simulink model "FixedWing_Model_nonlinearLQR_6_states"  (R2020b)
settings: Solver=VariableStepAuto  StartTime=0.0  StopTime=50  FixedStep=10^-4  RelTol=1e-7
values from neighbouring files (symbols this model uses):
  A_lat = [YB        Yp      -(u0-Yr)   g*cos(Theta0)   0;         A21       A22       A23        0             0;         A31       A32       A33        0             0;         0         1         0          0             0;         0         0         1          0             0]    [LQR_Dena_model_file_edited.m]
  A_long = [ Xu                    Xw              0              -g*cos(Theta0)            0;          Zu                    Zw              u0             -g*sin(Theta0)            0;          Mu+Mw_d*Zu            Mw+Mw_d*Zw      Mq+Mw_d*u0          0                    0;          0                     0               1                   0                    0;          -sin(Theta0)       -cos(Theta0)    ...(+51 chars)    [LQR_Dena_model_file_edited.m]
  b = 1.7    [LQR_Dena_model_file_edited.m]
  B_lat = [0        Ydr;        B21      B22;        B31      B32;        0        0;        0        0]    [LQR_Dena_model_file_edited.m]
  B_long = [ Xe         CXt;          Ze         0;          Me         0;          0          0;          0          0]    [LQR_Dena_model_file_edited.m]
  c = 0.28    [LQR_Dena_model_file_edited.m]
  C_lat = [0 0 0 1 0 ]    [LQR_Dena_model_file_edited.m]
  C_long = [0 0 0 1 0]    [LQR_Dena_model_file_edited.m]
  CL_aileron = 0.32935    [LQR_Dena_model_file_edited.m]
  CL_rudder = 0.003592    [LQR_Dena_model_file_edited.m]
  CLb = 0.029196    [LQR_Dena_model_file_edited.m]
  CLp = -0.44965    [LQR_Dena_model_file_edited.m]
  CLr = 0.0067709    [LQR_Dena_model_file_edited.m]
  CM_alpha = -0.1651    [LQR_Dena_model_file_edited.m]
  CM_alpha_dot = -6.5034    [LQR_Dena_model_file_edited.m]
  CMe = -1.3977    [LQR_Dena_model_file_edited.m]
  CMq = -11.7782    [LQR_Dena_model_file_edited.m]
  CMt = 0    [LQR_Dena_model_file_edited.m]
  CMu = 0.158*0    (= 0)    [LQR_Dena_model_file_edited.m]
  CN_aileron = 0.036215    [LQR_Dena_model_file_edited.m]
  CN_rudder = -0.045652    [LQR_Dena_model_file_edited.m]
  CNB = 0.066996    [LQR_Dena_model_file_edited.m]
  CNp = -0.030754    [LQR_Dena_model_file_edited.m]
  CNr = -0.064937    [LQR_Dena_model_file_edited.m]
  CX0 = -0.0094304    [LQR_Dena_model_file_edited.m]
  CX_alpha = (0.42565-0.21544)    (= 0.21021)    [LQR_Dena_model_file_edited.m]
  CXe = 0    [LQR_Dena_model_file_edited.m]
  CXt = 1    [LQR_Dena_model_file_edited.m]
  CXu = -(0.158*0)-0.0094304    (= -0.0094304)    [LQR_Dena_model_file_edited.m]
  CY_rudder = -0.10317    [LQR_Dena_model_file_edited.m]
  CYB = -0.16533    [LQR_Dena_model_file_edited.m]
  CYp = -0.00068802    [LQR_Dena_model_file_edited.m]
  CYr = 0.15502    [LQR_Dena_model_file_edited.m]
  CZ0 = -0.42565    [LQR_Dena_model_file_edited.m]
  CZ_alpha = -(4.8375+0.0094304)    (= -4.8469304)    [LQR_Dena_model_file_edited.m]
  CZ_alpha_dot = 1.3359    [LQR_Dena_model_file_edited.m]
  CZe = -0.56118    [LQR_Dena_model_file_edited.m]
  CZq = -7.3583    [LQR_Dena_model_file_edited.m]
  CZt = 0    [LQR_Dena_model_file_edited.m]
  CZu = -((0.052968^2)/(1-(0.052968)^2))*0.42565    (= -0.00119756738693)    [LQR_Dena_model_file_edited.m]
  d_aileron0 = 0    [LQR_Dena_model_file_edited.m]
  d_elevator0 = -0.6319*pi/180    (= -0.0110287355434)    [LQR_Dena_model_file_edited.m]
  D_long = zeros(5,2)    [LQR_Dena_model_file_edited.m]
  d_rudder0 = 0    [LQR_Dena_model_file_edited.m]
  d_Thrust0 = 5    [LQR_Dena_model_file_edited.m]
  e_longi = longd- [longi; 0]    [LQR_Dena_model_file_edited.m]
  Epsi0 = 0    [LQR_Dena_model_file_edited.m]
  Epsi_initial = Epsi0    (= 0)    [LQR_Dena_model_file_edited.m]
  g = 9.81    [LQR_Dena_model_file_edited.m]
  Hi = 120    [LQR_Dena_model_file_edited.m]
  Ix = 0.6465    [LQR_Dena_model_file_edited.m]
  Ixz = 0.0006584    [LQR_Dena_model_file_edited.m]
  Iy = 0.3048    [LQR_Dena_model_file_edited.m]
  Iz = 0.9359    [LQR_Dena_model_file_edited.m]
  K = K_long_hat(:,1:5)    [LQR_Dena_model_file_edited.m]
  K_lat_hat = lqr(A_lat_hat, B_lat_hat,Q_lat_hat,R_lat)    [LQR_Dena_model_file_edited.m]
  K_long = lqr(A_long, B_long,Q_long,R_long)    [LQR_Dena_model_file_edited.m]
  K_long_hat = lqr(A_long_hat, B_long_hat,Q_long_hat,R_long)    [LQR_Dena_model_file_edited.m]
  Ki = -K_long_hat(:,6)    [LQR_Dena_model_file_edited.m]
  lati = [ v_initial; p_initial; r_initial; Phi_initial; Epsi_initial]    [LQR_Dena_model_file_edited.m]
  longd = [u0; w0; q0; Theta0; Hi; 0]    [LQR_Dena_model_file_edited.m]
  longi = [ u_initial; w_initial; q_initial; Theta_initial; Ze0]    [LQR_Dena_model_file_edited.m]
  mass = 4    [LQR_Dena_model_file_edited.m]
  p0 = 0    [LQR_Dena_model_file_edited.m]
  p_initial = 0    [LQR_Dena_model_file_edited.m]
  Phi0 = 0    [LQR_Dena_model_file_edited.m]
  Phi_initial = Phi0    (= 0)    [LQR_Dena_model_file_edited.m]
  q0 = 0    [LQR_Dena_model_file_edited.m]
  q_initial = 0    [LQR_Dena_model_file_edited.m]
  r0 = 0    [LQR_Dena_model_file_edited.m]
  r_initial = 0    [LQR_Dena_model_file_edited.m]
  S = 0.471    [LQR_Dena_model_file_edited.m]
  Theta0 = 5.1*pi/180    (= 0.0890117918517)    [LQR_Dena_model_file_edited.m]
  Theta_initial = Theta0+(2*pi/180)    (= 0.123918376892)    [LQR_Dena_model_file_edited.m]
  u0 = sqrt(V0^2/(1+(tan(Theta0))^2))    [LQR_Dena_model_file_edited.m]
  u_initial = u0    [LQR_Dena_model_file_edited.m]
  v0 = 0    [LQR_Dena_model_file_edited.m]
  v_initial = v0    (= 0)    [LQR_Dena_model_file_edited.m]
  w0 = u0*tan(Theta0)    [LQR_Dena_model_file_edited.m]
  w_initial = w0    [LQR_Dena_model_file_edited.m]
  X0 = mass*g*sin(Theta0)    [LQR_Dena_model_file_edited.m]
  Xe0 = 0    [LQR_Dena_model_file_edited.m]
  Y0 = -mass*g*cos(Theta0)*sin(Phi0)    [LQR_Dena_model_file_edited.m]
  Ye0 = 0    [LQR_Dena_model_file_edited.m]
  Z0 = -mass*g*cos(Theta0)*cos(Phi0)    [LQR_Dena_model_file_edited.m]
  Ze0 = 120    [LQR_Dena_model_file_edited.m]
undefined symbols (not defined in the file or in its folder): A_hat, B_hat, C_hat, K_alt, K_e, Meu_e, use, W_e
libraries: simulink_extras x39, dspindex x3, aerolibatmos2 x1, aerolibutil x1, sharedtransform x1
(part 2 of 2)

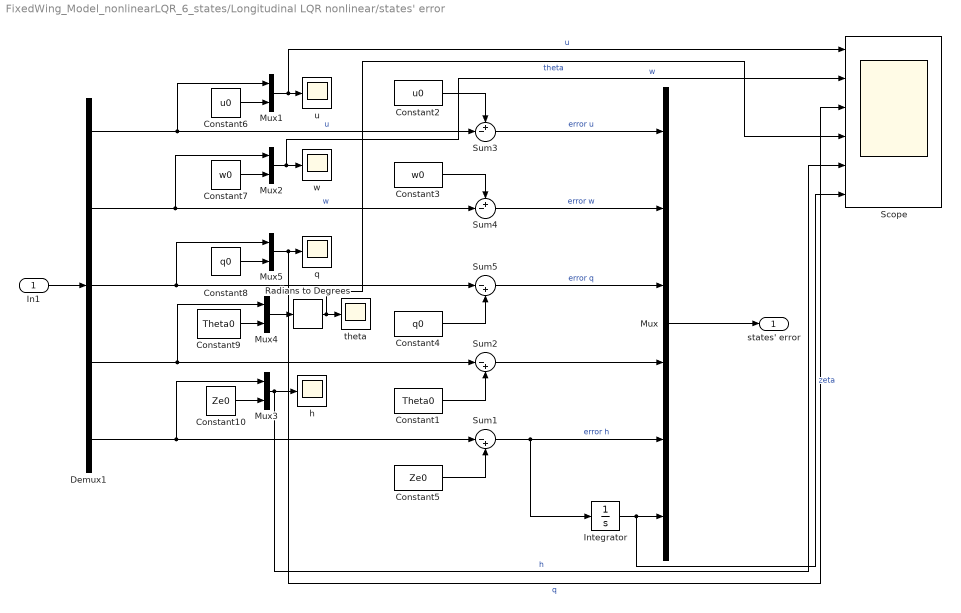
== system FixedWing_Model_nonlinearLQR_6_states/Longitudinal LQR nonlinear/states' error ==
  In1 : Inport
  Constant1 : Constant  Value=Theta0
  Constant10 : Constant  Value=Ze0
  Constant2 : Constant  Value=u0
  Constant3 : Constant  Value=w0
  Constant4 : Constant  Value=q0
  Constant5 : Constant  Value=Ze0
  Constant6 : Constant  Value=u0
  Constant7 : Constant  Value=w0
  Constant8 : Constant  Value=q0
  Constant9 : Constant  Value=Theta0
  Demux1 : Demux  Outputs=5
  Integrator : Integrator  InitialCondition=Ze0-Hi
  Mux : Mux  Inputs=6
  Mux{1..5} (5 alike) : Mux  Inputs=2
  Radians to Degrees : simulink_extras/Transformations/Radians to Degrees
  Scope : Scope  NumInputPorts=6
  Sum1 : Sum  Inputs=|-+
  Sum2 : Sum  Inputs=|-+
  Sum3 : Sum  Inputs=+-|
  Sum4 : Sum  Inputs=+-|
  Sum5 : Sum  Inputs=|-+
  h : Scope
  q : Scope
  theta : Scope
  u : Scope
  w : Scope
  states' error : Outport
  wires:
  Constant1/1 -> Sum2/2
  Constant4/1 -> Sum5/2
  Constant2/1 -> Sum3/1
  Sum3/1 -> Mux/1  "error u"
  Constant3/1 -> Sum4/1
  Sum4/1 -> Mux/2  "error w"
  In1/1 -> Demux1/1
  Sum5/1 -> Mux/3  "error q"
  Mux/1 -> states' error/1
  Constant5/1 -> Sum1/2
  Sum1/1 -> Mux/5, Integrator/1  "error h"
  Demux1/3 -> Mux5/1, Sum5/1
  Constant8/1 -> Mux5/2
  Constant9/1 -> Mux4/2
  Constant10/1 -> Mux3/2
  Constant7/1 -> Mux2/2
  Demux1/5 -> Mux3/1, Sum1/1
  Demux1/1 -> Mux1/1, Sum3/2  "u"
  Demux1/2 -> Mux2/1, Sum4/2  "w"
  Constant6/1 -> Mux1/2
  Mux1/1 -> Scope/1, u/1  "u"
  Mux2/1 -> Scope/2, w/1  "w"
  Mux5/1 -> Scope/3, q/1  "q"
  Mux3/1 -> Scope/5, h/1  "h"
  Demux1/4 -> Mux4/1, Sum2/1
  Mux4/1 -> Radians to Degrees/1
  Radians to Degrees/1 -> Scope/4, theta/1  "theta"
  Sum2/1 -> Mux/4
  Integrator/1 -> Scope/6, Mux/6  "zeta"

== system FixedWing_Model_nonlinearLQR_6_states/Longitudinal LQR nonlinear seperated/theta' error ==
  states : Inport
  Constant1 : Constant  Value=Theta0
  Constant10 : Constant  Value=Ze0
  Constant6 : Constant  Value=u0
  Constant7 : Constant  Value=w0
  Constant8 : Constant  Value=q0
  Constant9 : Constant  Value=Theta0
  Demux1 : Demux  Outputs=5
  Mux{1..4,6} (5 alike) : Mux  Inputs=2
  Radians to Degrees : simulink_extras/Transformations/Radians to Degrees
  Sum2 : Sum  Inputs=|-+
  h : Scope
  q : Scope
  theta : Scope
  u : Scope
  w : Scope
  theta' error : Outport
  wires:
  Constant1/1 -> Sum2/2
  states/1 -> Demux1/1
  Constant9/1 -> Mux4/2
  Demux1/4 -> Mux4/1, Sum2/1
  Mux4/1 -> Radians to Degrees/1
  Radians to Degrees/1 -> theta/1
  Sum2/1 -> theta' error/1
  Demux1/3 -> Mux6/1
  Mux2/1 -> w/1
  Mux3/1 -> h/1
  Demux1/1 -> Mux1/1
  Constant7/1 -> Mux2/2
  Constant8/1 -> Mux6/2
  Constant10/1 -> Mux3/2
  Mux1/1 -> u/1
  Mux6/1 -> q/1
  Demux1/5 -> Mux3/1
  Constant6/1 -> Mux1/2
  Demux1/2 -> Mux2/1

== system FixedWing_Model_nonlinearLQR_6_states/Non linear/Euler ==
  p : Inport
  q : Inport  Port=2
  r : Inport  Port=3
  Subsystem : Subsystem
  Subsystem1 : Subsystem
  Subsystem2 : Subsystem
  Phi : Outport
  Theta : Outport  Port=2
  epsi : Outport  Port=3
  wires:
  Subsystem1/1(Theta) -> Theta/1, [Theta]
  Subsystem2/1(epsi) -> epsi/1
  [q] -> Subsystem/2(q)
  Subsystem/1(Phi) -> Phi/1, [Phi]
  [Theta] -> Subsystem/3(Theta)
  [r] -> Subsystem1/2(r)
  [Phi] -> Subsystem1/3(Phi)
  [Theta] -> Subsystem2/3(Theta)
  [q] -> Subsystem2/2(q)
  p/1 -> [p]
  q/1 -> [q]
  r/1 -> [r]
  [p] -> Subsystem/1(p)
  [r] -> Subsystem/4(r)
  [q] -> Subsystem1/1(q)
  [r] -> Subsystem2/1(r)
  [Phi] -> Subsystem2/4(Phi)

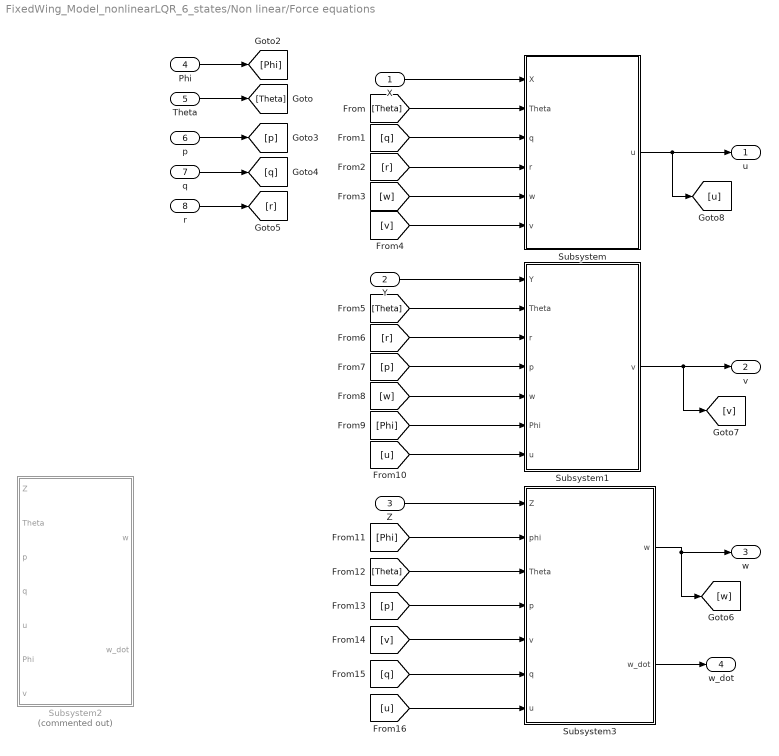
== system FixedWing_Model_nonlinearLQR_6_states/Non linear/Force equations ==
  X : Inport
  Y : Inport  Port=2
  Z : Inport  Port=3
  Phi : Inport  Port=4
  Theta : Inport  Port=5
  p : Inport  Port=6
  q : Inport  Port=7
  r : Inport  Port=8
  Subsystem : Subsystem
  Subsystem1 : Subsystem
  Subsystem2 : Subsystem  Commented=on
  Subsystem3 : Subsystem
  u : Outport
  v : Outport  Port=2
  w : Outport  Port=3
  w_dot : Outport  Port=4
  wires:
  Theta/1 -> [Theta]
  Phi/1 -> [Phi]
  p/1 -> [p]
  q/1 -> [q]
  r/1 -> [r]
  X/1 -> Subsystem/1(X)
  Y/1 -> Subsystem1/1(Y)
  Z/1 -> Subsystem3/1(Z)
  Subsystem/1(u) -> [u], u/1
  Subsystem1/1(v) -> v/1, [v]
  [Theta] -> Subsystem/2(Theta)
  [q] -> Subsystem/3(q)
  [r] -> Subsystem/4(r)
  [w] -> Subsystem/5(w)
  [v] -> Subsystem/6(v)
  [Theta] -> Subsystem1/2(Theta)
  [r] -> Subsystem1/3(r)
  [p] -> Subsystem1/4(p)
  [w] -> Subsystem1/5(w)
  [Phi] -> Subsystem1/6(Phi)
  [u] -> Subsystem1/7(u)
  [Phi] -> Subsystem3/2(phi)
  [p] -> Subsystem3/4(p)
  [v] -> Subsystem3/5(v)
  [q] -> Subsystem3/6(q)
  [u] -> Subsystem3/7(u)
  Subsystem3/1(w) -> [w], w/1
  Subsystem3/2(w_dot) -> w_dot/1
  [Theta] -> Subsystem3/3(Theta)

== system FixedWing_Model_nonlinearLQR_6_states/Non linear/Moment equations ==
  L : Inport
  M : Inport  Port=2
  N : Inport  Port=3
  Integrator : Integrator  InitialCondition=p_initial
  Integrator2 : Integrator  InitialCondition=r_initial
  Subsystem : Subsystem
  Subsystem1 : Subsystem
  Subsystem2 : Subsystem
  p : Outport
  q : Outport  Port=2
  r : Outport  Port=3
  wires:
  L/1 -> Subsystem/1(L)
  [r_dot] -> Subsystem/2(r_dot)
  [q] -> Subsystem/3(q)
  M/1 -> Subsystem1/1(M)
  Subsystem1/1(q) -> [q], q/1
  [p] -> Subsystem1/2(p)
  [r] -> Subsystem1/3(r)
  N/1 -> Subsystem2/1(N)
  [p] -> Subsystem2/2(p)
  [q] -> Subsystem2/3(q)
  [p_dot] -> Subsystem2/4(p_dot)
  Integrator/1 -> [p], p/1
  Subsystem/1(p_dot) -> [p_dot], Integrator/1
  [r] -> Subsystem/4(r)
  Integrator2/1 -> [r], r/1
  Subsystem2/1(r_dot) -> [r_dot], Integrator2/1

== system FixedWing_Model_nonlinearLQR_6_states/Non linear/transformation ==
  epsi : Inport
  u : Inport  Port=2
  v : Inport  Port=3
  w : Inport  Port=4
  Phi : Inport  Port=5
  Theta : Inport  Port=6
  Display : Display
      settings: Decimation=3
  Display1 : Display
  Display2 : Display
      settings: Decimation=3
  Integrator : Integrator  InitialCondition=Xe0
  Integrator1 : Integrator  InitialCondition=Ye0
  Integrator2 : Integrator  InitialCondition=Ze0
  Invert 3x3 Matrix : aerolibutil/Invert  3x3 Matrix
  MatrixMultiply : Product  Multiplication=Matrix(*)
  Mux : Mux  Inputs=3
  Mux1 : Mux  Inputs=3
  Reshape : Reshape  OutputDimensionality=Customize  OutputDimensions=1
  Reshape1 : Reshape  OutputDimensionality=Customize  OutputDimensions=1
  Reshape2 : Reshape  OutputDimensionality=Customize  OutputDimensions=1
  Rotation Angles to Direction Cosine Matrix : sharedtransform/Rotation Angles to Direction Cosine Matrix  rotationOrder=ZYX  aMode=aMode
      settings: SourceProductBaseCode=AE,PW,MT,UV,VE,VP
  Variable Selector : dspindex/Variable Selector  NumInputs=1  rowsOrCols=Rows  IdxMode=Fixed  Elements=[1]  ZerOneIdxMode=One-based  errmode=Clip Index  FillMode=on  FillValues=0
  Variable Selector1 : dspindex/Variable Selector  NumInputs=1  rowsOrCols=Rows  IdxMode=Fixed  Elements=[2]  ZerOneIdxMode=One-based  errmode=Clip Index  FillMode=on  FillValues=0
  Variable Selector2 : dspindex/Variable Selector  NumInputs=1  rowsOrCols=Rows  IdxMode=Fixed  Elements=[3]  ZerOneIdxMode=One-based  errmode=Clip Index  FillMode=on  FillValues=0
  X_position_dot : Outport
  Y_position_dot : Outport  Port=2
  Z_position_dot : Outport  Port=3
  X_position : Outport  Port=4
  Y_position : Outport  Port=5
  Z_position : Outport  Port=6
  wires:
  Rotation Angles to Direction Cosine Matrix/1 -> Invert 3x3 Matrix/1
  u/1 -> Mux/1
  v/1 -> Mux/2
  w/1 -> Mux/3
  Mux/1 -> Display2/1, MatrixMultiply/2
  Invert 3x3 Matrix/1 -> MatrixMultiply/1
  epsi/1 -> Mux1/1
  Theta/1 -> Mux1/2
  Phi/1 -> Mux1/3
  Mux1/1 -> Display/1, Rotation Angles to Direction Cosine Matrix/1
  MatrixMultiply/1 -> Variable Selector2/1, Variable Selector1/1, Variable Selector/1
  Variable Selector2/1 -> Reshape2/1
  Variable Selector1/1 -> Reshape1/1
  Variable Selector/1 -> Reshape/1
  Reshape/1 -> Integrator/1, X_position_dot/1
  Reshape1/1 -> Y_position_dot/1, Integrator1/1
  Reshape2/1 -> Display1/1, Integrator2/1, Z_position_dot/1
  Integrator/1 -> X_position/1
  Integrator1/1 -> Y_position/1
  Integrator2/1 -> Z_position/1

== system FixedWing_Model_nonlinearLQR_6_states/V and H/states' error ==
  In1 : Inport
  Constant1 : Constant  Value=Theta0
  Constant2 : Constant  Value=u0
  Constant3 : Constant  Value=w0
  Constant4 : Constant  Value=q0
  Demux1 : Demux
  Mux : Mux
  Radians to Degrees2 : simulink_extras/Transformations/Radians to Degrees
  Sum2 : Sum  Inputs=|-+
  Sum3 : Sum  Inputs=+-|
  Sum4 : Sum  Inputs=+-|
  Sum5 : Sum  Inputs=|-+
  q : Scope
  u : Scope
  w : Scope
  theta in degrees : Outport
  states' error : Outport  Port=2
  wires:
  Constant1/1 -> Sum2/2
  Demux1/2 -> Sum4/2, w/1
  Constant4/1 -> Sum5/2
  Sum2/1 -> Mux/4  "error theta"
  Constant2/1 -> Sum3/1
  Sum3/1 -> Mux/1  "error u"
  Constant3/1 -> Sum4/1
  Demux1/1 -> Sum3/2, u/1
  Demux1/3 -> Sum5/1, q/1
  Sum4/1 -> Mux/2  "error w"
  In1/1 -> Demux1/1
  Sum5/1 -> Mux/3  "error q"
  Mux/1 -> states' error/1
  Radians to Degrees2/1 -> theta in degrees/1
  Demux1/4 -> Radians to Degrees2/1, Sum2/1

== system FixedWing_Model_nonlinearLQR_6_states/linear paper/states' error1 ==
  In1 : Inport
  Constant1 : Constant  Value=Theta0
  Constant2 : Constant  Value=u0
  Constant3 : Constant  Value=w0
  Constant4 : Constant  Value=q0
  Demux1 : Demux
  Mux : Mux
  Scope : Scope
  Sum{1..4} (4 alike) : Sum  Inputs=-+|
  q : Scope
  u : Scope
  w : Scope
  states' error : Outport
  wires:
  Constant1/1 -> Sum4/1
  Demux1/2 -> Sum1/2, w/1
  Constant4/1 -> Sum2/1
  Demux1/4 -> Sum4/2
  Sum4/1 -> Scope/1, Mux/4  "error theta"
  Constant2/1 -> Sum3/1
  Sum3/1 -> Mux/1  "error u"
  Constant3/1 -> Sum1/1
  Demux1/1 -> Sum3/2, u/1
  Demux1/3 -> Sum2/2, q/1
  Sum1/1 -> Mux/2  "error w"
  In1/1 -> Demux1/1
  Sum2/1 -> Mux/3  "error q"
  Mux/1 -> states' error/1

== system FixedWing_Model_nonlinearLQR_6_states/Aerodynamic /Delta L moment/Subsystem ==
  r : Inport
  Q : Inport  Port=2
  (S*b^2)/(2*Ix*u0) : Gain  Gain=(S*b*b)/(2*Ix*u0)
  CLr : Gain  Gain=CLr
  Ix : Gain  Gain=Ix
  Product : Product
  Out1 : Outport
  wires:
  Q/1 -> (S*b^2)/(2*Ix*u0)/1
  Product/1 -> Out1/1
  CLr/1 -> Ix/1
  (S*b^2)/(2*Ix*u0)/1 -> CLr/1
  Ix/1 -> Product/1
  r/1 -> Product/2

== system FixedWing_Model_nonlinearLQR_6_states/Aerodynamic /Delta L moment/Subsystem1 ==
  rudder : Inport
  Q : Inport  Port=2
  (S*b)/(Ix) : Gain  Gain=(S*b)/(Ix)
  CL_rudder : Gain  Gain=CL_rudder
  Ix : Gain  Gain=Ix
  Product : Product
  Subtract : Sum  Inputs=+-
  d_rudder0 : Constant  Value=d_rudder0  VectorParams1D=off
  Out1 : Outport
  wires:
  Ix/1 -> Product/1
  (S*b)/(Ix)/1 -> CL_rudder/1
  Q/1 -> (S*b)/(Ix)/1
  Product/1 -> Out1/1
  CL_rudder/1 -> Ix/1
  d_rudder0/1 -> Subtract/2
  Subtract/1 -> Product/2  "delta_rudder"
  rudder/1 -> Subtract/1

== system FixedWing_Model_nonlinearLQR_6_states/Aerodynamic /Delta L moment/Subsystem2 ==
  aileron : Inport
  Q : Inport  Port=2
  (S*b)/(Ix) : Gain  Gain=(S*b)/(Ix)
  CL_aileron : Gain  Gain=CL_aileron
  Ix : Gain  Gain=Ix
  Product : Product
  Subtract : Sum  Inputs=+-
  d_aileron0 : Constant  Value=d_aileron0  VectorParams1D=off
  Out1 : Outport
  wires:
  (S*b)/(Ix)/1 -> CL_aileron/1
  CL_aileron/1 -> Ix/1
  Ix/1 -> Product/1
  d_aileron0/1 -> Subtract/2
  Product/1 -> Out1/1
  Subtract/1 -> Product/2  "delta_aileron"
  aileron/1 -> Subtract/1
  Q/1 -> (S*b)/(Ix)/1

== system FixedWing_Model_nonlinearLQR_6_states/Aerodynamic /Delta L moment/Subsystem3 ==
  p : Inport
  Q : Inport  Port=2
  (S*b^2)/(2*Ix*u0) : Gain  Gain=(S*b*b)/(2*Ix*u0)
  CLp : Gain  Gain=CLp
  Ix : Gain  Gain=Ix
  Product : Product
  Out1 : Outport
  wires:
  Ix/1 -> Product/1
  CLp/1 -> Ix/1
  (S*b^2)/(2*Ix*u0)/1 -> CLp/1
  Product/1 -> Out1/1
  p/1 -> Product/2
  Q/1 -> (S*b^2)/(2*Ix*u0)/1

== system FixedWing_Model_nonlinearLQR_6_states/Aerodynamic /Delta L moment/Subsystem4 ==
  v : Inport
  Q : Inport  Port=2
  (S*b)/(Ix*u0) : Gain  Gain=(S*b)/(Ix*u0)
  CLb : Gain  Gain=CLb
  Ix : Gain  Gain=Ix
  Product : Product
  Out1 : Outport
  wires:
  v/1 -> Product/2
  (S*b)/(Ix*u0)/1 -> CLb/1
  Ix/1 -> Product/1
  Q/1 -> (S*b)/(Ix*u0)/1
  Product/1 -> Out1/1
  CLb/1 -> Ix/1

== system FixedWing_Model_nonlinearLQR_6_states/Aerodynamic /Delta M moment/Subsystem ==
  w_dot : Inport
  Q : Inport  Port=2
  (S*c^2)/(2*Iy*u0^2) : Gain  Gain=(S*c*c)/(2*Iy*u0*u0)
  CM_alpha_dot : Gain  Gain=CM_alpha_dot
  Iy : Gain  Gain=Iy
  Product : Product
  Out1 : Outport
  wires:
  CM_alpha_dot/1 -> Iy/1
  (S*c^2)/(2*Iy*u0^2)/1 -> CM_alpha_dot/1
  w_dot/1 -> Product/2
  Q/1 -> (S*c^2)/(2*Iy*u0^2)/1
  Product/1 -> Out1/1
  Iy/1 -> Product/1

== system FixedWing_Model_nonlinearLQR_6_states/Aerodynamic /Delta M moment/Subsystem1 ==
  q : Inport
  Q : Inport  Port=2
  (S*c^2)/(2*Iy*u0) : Gain  Gain=(S*c*c)/(2*Iy*u0)
  CMq : Gain  Gain=CMq
  Iy : Gain  Gain=Iy
  Minus2 : Sum  Inputs=+-
  Product : Product
  q0 : Constant  Value=q0
  Out1 : Outport
  wires:
  Product/1 -> Out1/1
  Q/1 -> (S*c^2)/(2*Iy*u0)/1
  Iy/1 -> Product/1
  (S*c^2)/(2*Iy*u0)/1 -> CMq/1
  CMq/1 -> Iy/1
  q0/1 -> Minus2/2
  q/1 -> Minus2/1
  Minus2/1 -> Product/2

== system FixedWing_Model_nonlinearLQR_6_states/Aerodynamic /Delta M moment/Subsystem2 ==
  elevator : Inport
  Q : Inport  Port=2
  (S*c)/(Iy) : Gain  Gain=(S*c)/(Iy)
  CMe : Gain  Gain=CMe
  Iy : Gain  Gain=Iy
  Product1 : Product
  Subtract : Sum  Inputs=+-
  d_elevator0 : Constant  Value=d_elevator0  VectorParams1D=off
  Out3 : Outport
  wires:
  CMe/1 -> Iy/1
  (S*c)/(Iy)/1 -> CMe/1
  Iy/1 -> Product1/1
  Q/1 -> (S*c)/(Iy)/1
  Product1/1 -> Out3/1
  elevator/1 -> Subtract/1
  d_elevator0/1 -> Subtract/2
  Subtract/1 -> Product1/2  "delta_elevator"

== system FixedWing_Model_nonlinearLQR_6_states/Aerodynamic /Delta M moment/Subsystem3 ==
  w : Inport
  Q : Inport  Port=2
  (S*c)/(Iy*u0) : Gain  Gain=(S*c)/(Iy*u0)
  CM_alpha : Gain  Gain=CM_alpha
  Iy : Gain  Gain=Iy
  Minus1 : Sum  Inputs=+-
  Product : Product
  w0 : Constant  Value=w0
  Out1 : Outport
  wires:
  Product/1 -> Out1/1
  (S*c)/(Iy*u0)/1 -> CM_alpha/1
  Q/1 -> (S*c)/(Iy*u0)/1
  CM_alpha/1 -> Iy/1
  Iy/1 -> Product/1
  w/1 -> Minus1/1
  Minus1/1 -> Product/2
  w0/1 -> Minus1/2

== system FixedWing_Model_nonlinearLQR_6_states/Aerodynamic /Delta M moment/Subsystem4 ==
  u : Inport
  Q : Inport  Port=2
  (S*c)/(Iy*u0) : Gain  Gain=(S*c)/(Iy*u0)
  CMu : Gain  Gain=CMu
  Iy : Gain  Gain=Iy
  Minus : Sum  Inputs=+-
  Product : Product
  u0 : Constant  Value=u0
  Out1 : Outport
  wires:
  Iy/1 -> Product/1
  CMu/1 -> Iy/1
  (S*c)/(Iy*u0)/1 -> CMu/1
  Product/1 -> Out1/1
  Q/1 -> (S*c)/(Iy*u0)/1
  u0/1 -> Minus/2
  u/1 -> Minus/1
  Minus/1 -> Product/2

== system FixedWing_Model_nonlinearLQR_6_states/Aerodynamic /Delta M moment/Subsystem5 ==
  note: M_t=Q*S*CMt
  Thrust : Inport
  Q : Inport  Port=2
  CMt : Gain  Gain=CMt
  Product1 : Product
  S : Gain  Gain=S
  Subtract1 : Sum  Inputs=+-
  d_Thrust0 : Constant  Value=d_Thrust0
  Out1 : Outport
  wires:
  Product1/1 -> Out1/1
  d_Thrust0/1 -> Subtract1/2
  Q/1 -> S/1
  S/1 -> CMt/1
  Subtract1/1 -> Product1/2  "Delta_thrust"
  Thrust/1 -> Subtract1/1
  CMt/1 -> Product1/1

== system FixedWing_Model_nonlinearLQR_6_states/Aerodynamic /Delta N moment/Subsystem ==
  r : Inport
  Q : Inport  Port=2
  (S*b^2)/(2*Ix*u0) : Gain  Gain=(S*b*b)/(2*Ix*u0)
  CNr : Gain  Gain=CNr
  Ix : Gain  Gain=Ix
  Product : Product
  Out1 : Outport
  wires:
  r/1 -> Product/2
  Ix/1 -> Product/1
  Q/1 -> (S*b^2)/(2*Ix*u0)/1
  Product/1 -> Out1/1
  (S*b^2)/(2*Ix*u0)/1 -> CNr/1
  CNr/1 -> Ix/1

== system FixedWing_Model_nonlinearLQR_6_states/Aerodynamic /Delta N moment/Subsystem1 ==
  rudder : Inport
  Q : Inport  Port=2
  (S*b)/(Iz) : Gain  Gain=(S*b)/(Iz)
  CN_rudder : Gain  Gain=CN_rudder
  Iz : Gain  Gain=Iz
  Product : Product
  Subtract : Sum  Inputs=+-
  d_rudder0 : Constant  Value=d_rudder0  VectorParams1D=off
  Out1 : Outport
  wires:
  Q/1 -> (S*b)/(Iz)/1
  Iz/1 -> Product/1
  Subtract/1 -> Product/2  "delta_rudder"
  CN_rudder/1 -> Iz/1
  d_rudder0/1 -> Subtract/2
  (S*b)/(Iz)/1 -> CN_rudder/1
  rudder/1 -> Subtract/1
  Product/1 -> Out1/1

== system FixedWing_Model_nonlinearLQR_6_states/Aerodynamic /Delta N moment/Subsystem2 ==
  aileron : Inport
  Q : Inport  Port=2
  (S*b)/(Iz) : Gain  Gain=(S*b)/(Iz)
  CN_aileron : Gain  Gain=CN_aileron
  Iz : Gain  Gain=Iz
  Product : Product
  Subtract : Sum  Inputs=+-
  d_aileron0 : Constant  Value=d_aileron0  VectorParams1D=off
  Out1 : Outport
  wires:
  aileron/1 -> Subtract/1
  d_aileron0/1 -> Subtract/2
  Product/1 -> Out1/1
  (S*b)/(Iz)/1 -> CN_aileron/1
  CN_aileron/1 -> Iz/1
  Q/1 -> (S*b)/(Iz)/1
  Iz/1 -> Product/1
  Subtract/1 -> Product/2  "delta_aileron"

== system FixedWing_Model_nonlinearLQR_6_states/Aerodynamic /Delta N moment/Subsystem3 ==
  p : Inport
  Q : Inport  Port=2
  (S*b^2)/(2*Ix*u0) : Gain  Gain=(S*b*b)/(2*Ix*u0)
  CNp : Gain  Gain=CNp
  Ix : Gain  Gain=Ix
  Product : Product
  Out1 : Outport
  wires:
  CNp/1 -> Ix/1
  Ix/1 -> Product/1
  Q/1 -> (S*b^2)/(2*Ix*u0)/1
  p/1 -> Product/2
  (S*b^2)/(2*Ix*u0)/1 -> CNp/1
  Product/1 -> Out1/1

== system FixedWing_Model_nonlinearLQR_6_states/Aerodynamic /Delta N moment/Subsystem4 ==
  v : Inport
  Q : Inport  Port=2
  (S*b)/(Iz*u0) : Gain  Gain=(S*b)/(Iz*u0)
  CnB : Gain  Gain=CNB
  Iz : Gain  Gain=Iz
  Product : Product
  Out1 : Outport
  wires:
  Product/1 -> Out1/1
  v/1 -> Product/2
  Q/1 -> (S*b)/(Iz*u0)/1
  Iz/1 -> Product/1
  (S*b)/(Iz*u0)/1 -> CnB/1
  CnB/1 -> Iz/1

== system FixedWing_Model_nonlinearLQR_6_states/Aerodynamic /Delta X force/Subsystem ==
  Q : Inport
  u : Inport  Port=2
  2Cx0+Cxu : Gain  Gain=2*CX0+CXu
  Minus : Sum  Inputs=+-
  Product : Product
  S/(m*u0) : Gain  Gain=S/(mass*u0)
  m : Gain  Gain=mass
  u0 : Constant  Value=u0
  Out1 : Outport
  wires:
  Q/1 -> S/(m*u0)/1
  S/(m*u0)/1 -> 2Cx0+Cxu/1
  2Cx0+Cxu/1 -> m/1
  m/1 -> Product/1
  Product/1 -> Out1/1
  u0/1 -> Minus/2
  Minus/1 -> Product/2
  u/1 -> Minus/1

== system FixedWing_Model_nonlinearLQR_6_states/Aerodynamic /Delta X force/Subsystem1 ==
  Q : Inport
  w : Inport  Port=2
  CX_alpha : Gain  Gain=CX_alpha
  Minus1 : Sum  Inputs=+-
  Product : Product
  S/(mass*u0) : Gain  Gain=S/(mass*u0)
  m : Gain  Gain=mass
  w0 : Constant  Value=w0
  Out1 : Outport
  wires:
  Q/1 -> S/(mass*u0)/1
  S/(mass*u0)/1 -> CX_alpha/1
  Product/1 -> Out1/1
  Minus1/1 -> Product/2
  w/1 -> Minus1/1
  w0/1 -> Minus1/2
  CX_alpha/1 -> m/1
  m/1 -> Product/1

== system FixedWing_Model_nonlinearLQR_6_states/Aerodynamic /Delta X force/Subsystem2 ==
  note: X_e=Q*S*CXe
  Q : Inport
  elevator : Inport  Port=2
  CXe : Gain  Gain=CXe
  Product : Product
  S : Gain  Gain=S
  Subtract : Sum  Inputs=+-
  d_elevator0 : Constant  Value=d_elevator0  VectorParams1D=off
  Out1 : Outport
  wires:
  Q/1 -> S/1
  Product/1 -> Out1/1
  S/1 -> CXe/1
  CXe/1 -> Product/1
  elevator/1 -> Subtract/1
  d_elevator0/1 -> Subtract/2
  Subtract/1 -> Product/2  "delta_elevator"

== system FixedWing_Model_nonlinearLQR_6_states/Aerodynamic /Delta X force/Subsystem3 ==
  note: X_t=Q*S*CXt
  Q : Inport
  Thrust : Inport  Port=2
  CXt : Gain  Gain=CXt
  Product : Product
  S : Gain  Gain=S
  Subtract : Sum  Inputs=+-
  d_Thrust0 : Constant  Value=d_Thrust0
  Out2 : Outport
  wires:
  S/1 -> CXt/1
  Product/1 -> Out2/1
  Q/1 -> S/1
  CXt/1 -> Product/1
  Thrust/1 -> Subtract/1
  Subtract/1 -> Product/2  "Delta_thrust"
  d_Thrust0/1 -> Subtract/2

== system FixedWing_Model_nonlinearLQR_6_states/Aerodynamic /Delta Z force/Subsystem ==
  w : Inport
  Q : Inport  Port=2
  CZ_alpha : Gain  Gain=CZ_alpha
  Minus1 : Sum  Inputs=+-
  Product : Product
  S/(m*u0) : Gain  Gain=S/(mass*u0)
  m : Gain  Gain=mass
  w0 : Constant  Value=w0
  Out2 : Outport
  wires:
  Product/1 -> Out2/1
  CZ_alpha/1 -> m/1
  m/1 -> Product/1
  Q/1 -> S/(m*u0)/1
  S/(m*u0)/1 -> CZ_alpha/1
  Minus1/1 -> Product/2
  w/1 -> Minus1/1
  w0/1 -> Minus1/2

== system FixedWing_Model_nonlinearLQR_6_states/Aerodynamic /Delta Z force/Subsystem1 ==
  w_dot : Inport
  Q : Inport  Port=2
  (S*c)/(2m*u0^2) : Gain  Gain=(S*c)/(2*mass*u0*u0)
  CZ_alpha_dot : Gain  Gain=CZ_alpha_dot
  Product : Product
  m : Gain  Gain=mass
  Out2 : Outport
  wires:
  (S*c)/(2m*u0^2)/1 -> CZ_alpha_dot/1
  m/1 -> Product/1
  w_dot/1 -> Product/2
  Q/1 -> (S*c)/(2m*u0^2)/1
  Product/1 -> Out2/1
  CZ_alpha_dot/1 -> m/1

== system FixedWing_Model_nonlinearLQR_6_states/Aerodynamic /Delta Z force/Subsystem2 ==
  q : Inport
  Q : Inport  Port=2
  (S*c)/(2m*u0) : Gain  Gain=(S*c)/(2*mass*u0)
  CZq : Gain  Gain=CZq
  Minus2 : Sum  Inputs=+-
  Product : Product
  m : Gain  Gain=mass
  q0 : Constant  Value=q0
  Out1 : Outport
  wires:
  CZq/1 -> m/1
  Product/1 -> Out1/1
  Q/1 -> (S*c)/(2m*u0)/1
  m/1 -> Product/1
  (S*c)/(2m*u0)/1 -> CZq/1
  Minus2/1 -> Product/2
  q/1 -> Minus2/1
  q0/1 -> Minus2/2

== system FixedWing_Model_nonlinearLQR_6_states/Aerodynamic /Delta Z force/Subsystem3 ==
  note: done without (-) sign
  elevator : Inport
  Q : Inport  Port=2
  CZe : Gain  Gain=CZe
  Product : Product
  S/m : Gain  Gain=S/mass
  Subtract : Sum  Inputs=+-
  d_elevator0 : Constant  Value=d_elevator0  VectorParams1D=off
  m : Gain  Gain=mass
  Out1 : Outport
  wires:
  Subtract/1 -> Product/2  "delta_elevator"
  Product/1 -> Out1/1
  elevator/1 -> Subtract/1
  S/m/1 -> CZe/1
  d_elevator0/1 -> Subtract/2
  Q/1 -> S/m/1
  CZe/1 -> m/1
  m/1 -> Product/1

== system FixedWing_Model_nonlinearLQR_6_states/Aerodynamic /Delta Z force/Subsystem4 ==
  u : Inport
  Q : Inport  Port=2
  2*CZ0+CZu : Gain  Gain=2*CZ0+CZu
  Minus : Sum  Inputs=+-
  Product : Product
  S/(m*u0) : Gain  Gain=S/(mass*u0)
  m : Gain  Gain=mass
  u0 : Constant  Value=u0
  Out2 : Outport
  wires:
  S/(m*u0)/1 -> 2*CZ0+CZu/1
  m/1 -> Product/1
  Q/1 -> S/(m*u0)/1
  Product/1 -> Out2/1
  2*CZ0+CZu/1 -> m/1
  u0/1 -> Minus/2
  Minus/1 -> Product/2
  u/1 -> Minus/1

== system FixedWing_Model_nonlinearLQR_6_states/Aerodynamic /Delta Z force/Subsystem6 ==
  note: Z_t=Q*S*CZt
  Thrust : Inport
  Q : Inport  Port=2
  CZt : Gain  Gain=CZt
  Product : Product
  S : Gain
  Subtract : Sum  Inputs=+-
  d_Thrust0 : Constant  Value=d_Thrust0
  Out1 : Outport
  wires:
  Subtract/1 -> Product/2  "Delta_thrust"
  S/1 -> CZt/1
  d_Thrust0/1 -> Subtract/2
  Q/1 -> S/1
  Product/1 -> Out1/1
  Thrust/1 -> Subtract/1
  CZt/1 -> Product/1

== system FixedWing_Model_nonlinearLQR_6_states/Aerodynamic /DeltaY force/Subsystem ==
  note: Yv=YB/u0
  v : Inport
  Q : Inport  Port=2
  CYB : Gain  Gain=CYB
  Product : Product
  S/(m*u0) : Gain  Gain=S/(mass*u0)
  m : Gain  Gain=mass
  Out1 : Outport
  wires:
  Q/1 -> S/(m*u0)/1
  S/(m*u0)/1 -> CYB/1
  CYB/1 -> m/1
  m/1 -> Product/1
  v/1 -> Product/2
  Product/1 -> Out1/1

== system FixedWing_Model_nonlinearLQR_6_states/Aerodynamic /DeltaY force/Subsystem1 ==
  p : Inport
  Q : Inport  Port=2
  (S*b)/(2*mass*u0) : Gain  Gain=(S*b)/(2*mass*u0)
  CYp : Gain  Gain=CYp
  Product : Product
  m : Gain  Gain=mass
  Out2 : Outport
  wires:
  Product/1 -> Out2/1
  p/1 -> Product/2
  CYp/1 -> m/1
  (S*b)/(2*mass*u0)/1 -> CYp/1
  Q/1 -> (S*b)/(2*mass*u0)/1
  m/1 -> Product/1

== system FixedWing_Model_nonlinearLQR_6_states/Aerodynamic /DeltaY force/Subsystem2 ==
  r : Inport
  Q : Inport  Port=2
  (S*b)/(2*mass*u0) : Gain  Gain=(S*b)/(2*mass*u0)
  CYr : Gain  Gain=CYr
  Product : Product
  m : Gain  Gain=mass
  Out2 : Outport
  wires:
  CYr/1 -> m/1
  Q/1 -> (S*b)/(2*mass*u0)/1
  (S*b)/(2*mass*u0)/1 -> CYr/1
  Product/1 -> Out2/1
  r/1 -> Product/2
  m/1 -> Product/1

== system FixedWing_Model_nonlinearLQR_6_states/Aerodynamic /DeltaY force/Subsystem3 ==
  rudder : Inport
  Q : Inport  Port=2
  CY_rudder : Gain  Gain=CY_rudder
  Product : Product
  S/m : Gain  Gain=S/mass
  Subtract : Sum  Inputs=+-
  d_rudder0 : Constant  Value=d_rudder0
  m : Gain  Gain=mass
  Out1 : Outport
  wires:
  Q/1 -> S/m/1
  S/m/1 -> CY_rudder/1
  Product/1 -> Out1/1
  rudder/1 -> Subtract/1
  d_rudder0/1 -> Subtract/2
  Subtract/1 -> Product/2  "delta_rudder"
  CY_rudder/1 -> m/1
  m/1 -> Product/1

== system FixedWing_Model_nonlinearLQR_6_states/Longitudinal LQR elevator &thrust/all system/states' error ==
  In1 : Inport
  Constant1 : Constant  Value=Theta0
  Constant2 : Constant  Value=u0
  Constant3 : Constant  Value=w0
  Constant4 : Constant  Value=q0
  Demux1 : Demux
  Mux : Mux
  Radians to Degrees2 : simulink_extras/Transformations/Radians to Degrees
  Sum2 : Sum  Inputs=|-+
  Sum3 : Sum  Inputs=+-|
  Sum4 : Sum  Inputs=+-|
  Sum5 : Sum  Inputs=|-+
  q : Scope
  u : Scope
  w : Scope
  theta in degrees : Outport
  states' error : Outport  Port=2
  wires:
  Constant1/1 -> Sum2/2
  Demux1/2 -> Sum4/2, w/1
  Constant4/1 -> Sum5/2
  Demux1/4 -> Sum2/1, Radians to Degrees2/1
  Sum2/1 -> Mux/4  "error theta"
  Constant2/1 -> Sum3/1
  Sum3/1 -> Mux/1  "error u"
  Constant3/1 -> Sum4/1
  Demux1/1 -> Sum3/2, u/1
  Demux1/3 -> Sum5/1, q/1
  Sum4/1 -> Mux/2  "error w"
  In1/1 -> Demux1/1
  Sum5/1 -> Mux/3  "error q"
  Mux/1 -> states' error/1
  Radians to Degrees2/1 -> theta in degrees/1

== system FixedWing_Model_nonlinearLQR_6_states/Longitudinal LQR elevator only/all system/states' error ==
  In1 : Inport
  Constant1 : Constant  Value=Theta0
  Constant2 : Constant  Value=u_initial
  Constant3 : Constant  Value=w_initial
  Constant4 : Constant  Value=q_initial
  Demux1 : Demux
  Mux : Mux
  Radians to Degrees2 : simulink_extras/Transformations/Radians to Degrees
  Sum2 : Sum  Inputs=|-+
  Sum3 : Sum  Inputs=+-|
  Sum4 : Sum  Inputs=+-|
  Sum5 : Sum  Inputs=|-+
  q : Scope
  u : Scope
  w : Scope
  theta in degrees : Outport
  states' error : Outport  Port=2
  wires:
  Constant1/1 -> Sum2/2
  Demux1/2 -> w/1, Sum4/2
  Constant4/1 -> Sum5/2
  Demux1/4 -> Radians to Degrees2/1, Sum2/1
  Sum2/1 -> Mux/4  "error theta"
  Constant2/1 -> Sum3/1
  Sum3/1 -> Mux/1  "error u"
  Constant3/1 -> Sum4/1
  Demux1/1 -> u/1, Sum3/2
  Demux1/3 -> q/1, Sum5/1
  Sum4/1 -> Mux/2  "error w"
  In1/1 -> Demux1/1
  Sum5/1 -> Mux/3  "error q"
  Mux/1 -> states' error/1
  Radians to Degrees2/1 -> theta in degrees/1

== system FixedWing_Model_nonlinearLQR_6_states/Longitudinal LQR elevator only/states from ss/states' error ==
  In1 : Inport
  Constant1 : Constant  Value=Theta0
  Constant2 : Constant  Value=u_initial
  Constant3 : Constant  Value=w_initial
  Constant4 : Constant  Value=q_initial
  Demux1 : Demux
  Mux : Mux
  Radians to Degrees2 : simulink_extras/Transformations/Radians to Degrees
  Sum2 : Sum  Inputs=|+-
  Sum3 : Sum  Inputs=-+|
  Sum4 : Sum  Inputs=-+|
  Sum5 : Sum  Inputs=|+-
  theta in degrees : Outport
  states' error : Outport  Port=2
  wires:
  Constant1/1 -> Sum2/2
  Demux1/2 -> Sum4/2
  Constant4/1 -> Sum5/2
  Demux1/4 -> Radians to Degrees2/1, Sum2/1
  Sum2/1 -> Mux/4  "error theta"
  Constant2/1 -> Sum3/1
  Sum3/1 -> Mux/1  "error u"
  Constant3/1 -> Sum4/1
  Demux1/1 -> Sum3/2
  Demux1/3 -> Sum5/1
  Sum4/1 -> Mux/2  "error w"
  In1/1 -> Demux1/1
  Sum5/1 -> Mux/3  "error q"
  Mux/1 -> states' error/1
  Radians to Degrees2/1 -> theta in degrees/1

== system FixedWing_Model_nonlinearLQR_6_states/Non linear/Euler/Subsystem ==
  p : Inport
  q : Inport  Port=2
  Theta : Inport  Port=3
  r : Inport  Port=4
  Add : Sum  Inputs=+++
  Display : Display
  Integrator : Integrator  InitialCondition=Phi_initial
  Product : Product  Inputs=3
  Product1 : Product  Inputs=3
  Sin : Trigonometry  Operator=tan
  Sin1 : Trigonometry
  Sin3 : Trigonometry  Operator=cos
  Phi : Outport
  wires:
  Integrator/1 -> [Phi], Display/1, Phi/1
  q/1 -> Product/1
  Add/1 -> Integrator/1  "Phi_dot"
  Theta/1 -> Sin/1
  Sin/1 -> Product/2, Product1/2
  [Phi] -> Sin1/1
  Sin1/1 -> Product/3
  [Phi] -> Sin3/1
  r/1 -> Product1/1
  Sin3/1 -> Product1/3
  Product1/1 -> Add/3
  Product/1 -> Add/1
  p/1 -> Add/2

== system FixedWing_Model_nonlinearLQR_6_states/Non linear/Euler/Subsystem1 ==
  q : Inport
  r : Inport  Port=2
  Phi : Inport  Port=3
  Add : Sum  Inputs=+-
  Cos1 : Trigonometry
  Display : Display
  Integrator1 : Integrator  InitialCondition=Theta_initial
  Product : Product
  Product1 : Product
  Sin : Trigonometry  Operator=cos
  Theta : Outport
  wires:
  Add/1 -> Integrator1/1  "Theta_dot"
  Product/1 -> Add/2
  r/1 -> Product/1
  Integrator1/1 -> Display/1, Theta/1
  Phi/1 -> Cos1/1, Sin/1
  Cos1/1 -> Product/2
  Sin/1 -> Product1/2
  Product1/1 -> Add/1
  q/1 -> Product1/1

== system FixedWing_Model_nonlinearLQR_6_states/Non linear/Euler/Subsystem2 ==
  r : Inport
  q : Inport  Port=2
  Theta : Inport  Port=3
  Phi : Inport  Port=4
  Add : Sum
  Cos : Trigonometry  Operator=cos
  Cos1 : Trigonometry  Operator=cos
  Integrator2 : Integrator  InitialCondition=Epsi_initial
  Product : Product
  Product1 : Product
  Product3 : Product
  Reciprocal : Product  Inputs=/
  Sin : Trigonometry
  epsi : Outport
  wires:
  [Phi] -> Sin/1
  Product/1 -> Add/2
  q/1 -> Product/1
  Add/1 -> Product1/1
  Product1/1 -> Integrator2/1  "epsi_dot"
  Sin/1 -> Product/2
  Theta/1 -> Cos1/1
  Cos1/1 -> Reciprocal/1
  Reciprocal/1 -> Product1/2
  Product3/1 -> Add/1
  r/1 -> Product3/1
  Phi/1 -> [Phi]
  [Phi] -> Cos/1
  Cos/1 -> Product3/2
  Integrator2/1 -> epsi/1

== system FixedWing_Model_nonlinearLQR_6_states/Non linear/Force equations/Subsystem ==
  X : Inport
  Theta : Inport  Port=2
  q : Inport  Port=3
  r : Inport  Port=4
  w : Inport  Port=5
  v : Inport  Port=6
  1/m : Gain  Gain=1/mass
  Add : Sum  Inputs=+-
  Add1 : Sum  Inputs=++-
  Display : Display
  Display1 : Display
  Display2 : Display
  Integrator : Integrator  InitialCondition=u_initial
  Product : Product
  Product1 : Product
  Sin : Trigonometry
  m*g : Gain  Gain=mass*g
  u : Outport
  wires:
  Integrator/1 -> u/1
  Add1/1 -> Integrator/1  "u_dot"
  Theta/1 -> Sin/1
  X/1 -> Add/1
  Add/1 -> 1/m/1
  1/m/1 -> Display/1, Add1/1
  Sin/1 -> m*g/1
  m*g/1 -> Add/2
  r/1 -> Product1/1
  v/1 -> Product1/2
  Product1/1 -> Display1/1, Add1/2
  q/1 -> Product/1
  w/1 -> Product/2
  Product/1 -> Add1/3, Display2/1

== system FixedWing_Model_nonlinearLQR_6_states/Non linear/Force equations/Subsystem1 ==
  Y : Inport
  Theta : Inport  Port=2
  r : Inport  Port=3
  p : Inport  Port=4
  w : Inport  Port=5
  Phi : Inport  Port=6
  u : Inport  Port=7
  1/m : Gain  Gain=1/mass
  Add : Sum
  Add1 : Sum  Inputs=++-
  Integrator1 : Integrator  InitialCondition=v_initial
  Product : Product
  Product1 : Product
  Product2 : Product
  cos : Trigonometry  Operator=cos
  m*g : Gain  Gain=mass*g
  sin : Trigonometry
  v : Outport
  wires:
  Add1/1 -> Integrator1/1  "v_dot"
  w/1 -> Product1/2
  Product1/1 -> Add1/2
  p/1 -> Product1/1
  Add/1 -> 1/m/1
  cos/1 -> m*g/1
  Theta/1 -> cos/1
  Product/1 -> Add1/3
  Y/1 -> Add/1
  r/1 -> Product/1
  1/m/1 -> Add1/1
  Integrator1/1 -> v/1
  Product2/1 -> Add/2
  m*g/1 -> Product2/1
  Phi/1 -> sin/1
  sin/1 -> Product2/2
  u/1 -> Product/2

== system FixedWing_Model_nonlinearLQR_6_states/Non linear/Force equations/Subsystem2 ==
  Z : Inport
  Theta : Inport  Port=2
  p : Inport  Port=3
  q : Inport  Port=4
  u : Inport  Port=5
  Phi : Inport  Port=6
  v : Inport  Port=7
  1/m : Gain  Gain=1/mass
  Add : Sum
  Add1 : Sum  Inputs=++-
  Integrator2 : Integrator  InitialCondition=w_initial
  Product : Product
  Product1 : Product
  Product2 : Product
  c : Trigonometry  Operator=cos
  cos : Trigonometry  Operator=cos
  m*g : Gain  Gain=mass*g
  w : Outport
  w_dot : Outport  Port=2
  wires:
  Integrator2/1 -> w/1
  Add1/1 -> w_dot/1, Integrator2/1  "w_dot"
  Product/1 -> Add1/3
  1/m/1 -> Add1/1
  p/1 -> Product/1
  Product2/1 -> Add/2
  m*g/1 -> Product2/1
  Theta/1 -> cos/1
  cos/1 -> m*g/1
  q/1 -> Product1/1
  c/1 -> Product2/2
  u/1 -> Product1/2
  Z/1 -> Add/1
  Phi/1 -> c/1
  Product1/1 -> Add1/2
  Add/1 -> 1/m/1
  v/1 -> Product/2

== system FixedWing_Model_nonlinearLQR_6_states/Non linear/Force equations/Subsystem3 ==
  Z : Inport
  phi : Inport  Port=2
  Theta : Inport  Port=3
  p : Inport  Port=4
  v : Inport  Port=5
  q : Inport  Port=6
  u : Inport  Port=7
  1/m : Gain  Gain=1/mass
  Add : Sum  Inputs=+-+
  Add1 : Sum
  Cos : Trigonometry  Operator=cos
  Integrator : Integrator  InitialCondition=w_initial
  Product : Product
  Product1 : Product
  Product2 : Product
  Sin : Trigonometry  Operator=cos
  m*g : Gain  Gain=mass*g
  w : Outport
  w_dot : Outport  Port=2
  wires:
  Add1/1 -> 1/m/1
  1/m/1 -> Add/1
  Z/1 -> Add1/1
  m*g/1 -> Add1/2
  Product/1 -> m*g/1
  Sin/1 -> Product/1
  Cos/1 -> Product/2
  phi/1 -> Sin/1
  Theta/1 -> Cos/1
  Product1/1 -> Add/2
  p/1 -> Product1/1
  v/1 -> Product1/2
  q/1 -> Product2/1
  u/1 -> Product2/2
  Product2/1 -> Add/3
  Add/1 -> w_dot/1, Integrator/1
  Integrator/1 -> w/1

== system FixedWing_Model_nonlinearLQR_6_states/Non linear/Moment equations/Subsystem ==
  L : Inport
  r_dot : Inport  Port=2
  q : Inport  Port=3
  r : Inport  Port=4
  1/Ix : Gain  Gain=1/Ix
  Add : Sum  Inputs=+++-
  Gain : Gain  Gain=Ixz
  Gain1 : Gain  Gain=Ixz
  Integrator1 : Integrator  InitialCondition=p_initial
  Iz-Iy : Gain  Gain=Iz-Iy
  Product : Product
  Product1 : Product
  p_dot : Outport
  wires:
  L/1 -> Add/1
  Gain/1 -> Add/2
  q/1 -> Product/2, Product1/1
  Add/1 -> 1/Ix/1
  Product/1 -> Gain1/1
  Gain1/1 -> Add/3
  Product1/1 -> Iz-Iy/1
  r_dot/1 -> Gain/1
  1/Ix/1 -> Integrator1/1, p_dot/1
  Iz-Iy/1 -> Add/4
  Integrator1/1 -> [p]
  [p] -> Product/1
  r/1 -> Product1/2

== system FixedWing_Model_nonlinearLQR_6_states/Non linear/Moment equations/Subsystem1 ==
  M : Inport
  p : Inport  Port=2
  r : Inport  Port=3
  1/Iy : Gain  Gain=1/Iy
  Add : Sum  Inputs=+--
  Add1 : Sum  Inputs=+-
  Display : Display
  Display1 : Display
  Gain : Gain  Gain=Ixz
  Integrator1 : Integrator  InitialCondition=q_initial
  Ix-Iz : Gain  Gain=Ix-Iz
  Product1 : Product
  Square : Math  Operator=square  SaturateOnIntegerOverflow=on
  Square1 : Math  Operator=square  SaturateOnIntegerOverflow=on
  q : Outport
  wires:
  Integrator1/1 -> q/1, [q]
  Add/1 -> 1/Iy/1
  Product1/1 -> Ix-Iz/1
  1/Iy/1 -> Display/1, Integrator1/1  "q_dot"
  M/1 -> Display1/1, Add/1
  [q] -> Product1/2
  Ix-Iz/1 -> Add/3
  Add1/1 -> Gain/1
  p/1 -> Square/1
  Square/1 -> Add1/1
  r/1 -> Product1/1, Square1/1  "r"
  Square1/1 -> Add1/2
  Gain/1 -> Add/2

== system FixedWing_Model_nonlinearLQR_6_states/Non linear/Moment equations/Subsystem2 ==
  N : Inport
  p : Inport  Port=2
  q : Inport  Port=3
  p_dot : Inport  Port=4
  (Ixz) : Gain  Gain=Ixz
  1/Iz : Gain  Gain=1/Iz
  Add : Sum  Inputs=++--
  Integrator2 : Integrator  InitialCondition=r_initial
  Ixz : Gain  Gain=Ixz
  Iy-Ix : Gain  Gain=Iy-Ix
  Product1 : Product
  Product2 : Product
  r_dot : Outport
  wires:
  1/Iz/1 -> Integrator2/1, r_dot/1  "r_dot"
  Product2/1 -> Iy-Ix/1
  N/1 -> Add/1
  Add/1 -> 1/Iz/1
  p/1 -> Product2/1
  Product1/1 -> (Ixz)/1
  Ixz/1 -> Add/2
  p_dot/1 -> Ixz/1
  q/1 -> Product1/1, Product2/2
  Iy-Ix/1 -> Add/3
  [r] -> Product1/2
  (Ixz)/1 -> Add/4
  Integrator2/1 -> [r]
